simulink library "SimscapeUDP"  (R2020a)
settings: Solver=VariableStepAuto  StartTime=0.0  StopTime=10.0  RelTol=1e-3
libraries: dspnetwork x2, $bdroot x1
settings Model: Creator=cameron  LastModifiedBy=cameron

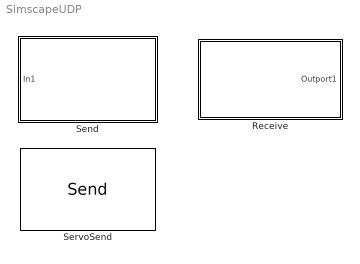
== system SimscapeUDP ==
  Receive : Subsystem  mask(ProtobufReceive){LocalPort=5002}
      mask help:
      | Revices Data on the Local Port.
      |
      | Outputs data as a Vector Width width real array representing the Servo Target Positions
      mask init:
      | set_param([gcb '/UDP Receive'], 'LocalPort', get_param(gcb,'LocalPort'));
      mask Help:
      | Input:
      | 	A searilised  protobuf object sent over UDP to the LocalPort.
      | 
      | Output:
      | 	A Vector Width width real array representing the Servo Target Positions.
      mask Display: disp(['LocalPort: ' get_param(gcb,'LocalPort') '\n\n']);
  Send : Subsystem  mask(ProtobufSend){IP='127.0.0.1', RemotePort=5002}
      mask help: Sends data to Remote Port at IP.
      mask init:
      | set_param([gcb '/UDP Send'], 'remoteURL', get_param(gcb,'ip'));
      | set_param([gcb '/UDP Send'], 'remotePort', get_param(gcb,'RemotePort'));
      mask Help:
      | Inputs:
      | 	DarwinSensors bus
      | 
      | Outpus:
      | 	Sends the array using protobuf to the given remote port.
      mask Display:
      | disp(['IP: ' get_param(gcb,'ip') '\n\n']);
      | disp(['RemotePort: ' get_param(gcb,'RemotePort')]);
  ServoSend : $bdroot/Send  IP='127.0.0.1'  RemotePort=5002
      link override S-Function: FunctionName=SfunProtobufServosEncode

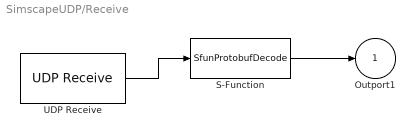
== system SimscapeUDP/Receive ==
  S-Function : S-Function  FunctionName=SfunProtobufDecode  SFunctionDeploymentMode=off  EnableBusSupport=off
  UDP Receive : dspnetwork/UDP Receive  localURL='0.0.0.0'  localPort=5002  remoteURL='0.0.0.0'  remotePort=-1  recvBufferSize=8192  dims=512  signalDatatype=uint8  isComplex=off  isVarSize=on  showBlockingTime=off  blockingTime=0  sampletime=0.1  blockPlatform=[]
  Outport1 : Outport  OutDataTypeStr=Bus: ServoTargetsBus
  wires:
  S-Function/1 -> Outport1/1
  UDP Receive/1 -> S-Function/1

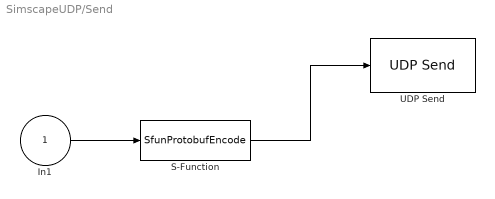
== system SimscapeUDP/Send ==
  In1 : Inport  OutDataTypeStr=Bus: DarwinSensorsBus  PortDimensions=1
  S-Function : S-Function  FunctionName=SfunProtobufEncode  SFunctionDeploymentMode=off  EnableBusSupport=off
  UDP Send : dspnetwork/UDP Send  remoteURL='127.0.0.1'  remotePort=5002  localURL='0.0.0.0'  localPortSource=Automatically determine  localPort=2048  sendBufferSize=8192  sampletime=-1  blockPlatform=[]  separateLengthPort=0
  wires:
  In1/1 -> S-Function/1
  S-Function/1 -> UDP Send/1
